simulink model "OPLOOP"  (Simulink 3.00)
settings: Solver=ode45  StartTime=0.0  StopTime=400.0  RelTol=1e-3
libraries: simulink3 x2

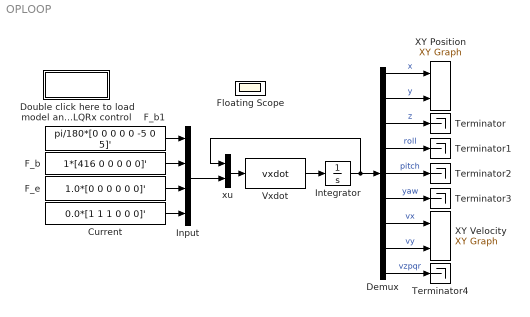
== system OPLOOP ==
  Current : Constant  Value=0.0*[1 1 1 0 0 0]'
  Demux : Demux  Outputs=[1 1 1 1 1 1 1 1 4]
  "Double click here to load model and  LQRx control " : Subsystem
      settings: OpenFcn=shark;global veh;[v1,veh,v3]=vehicle;
      mask Display: disp('Load Data')
  F_b : Constant  Value=1*[416 0 0 0 0 0]'
  F_b1 : Constant  Value=pi/180*[0 0 0 0 0 -5 0 5]'
  F_e : Constant  Value=1.0*[0 0 0 0 0 0]'
  Floating Scope : Scope
      settings: Floating=on  TimeRange=auto  YMin=-1  YMax=1  SaveToWorkspace=off  SaveName=ScopeData  LimitMaxRows=off
  Input : Mux  Inputs=[8 6 6 6]
  Integrator : Integrator  ExternalReset=none  InitialConditionSource=internal  InitialCondition=0  LimitOutput=off  UpperSaturationLimit=inf  LowerSaturationLimit=-inf  ShowSaturationPort=off  ShowStatePort=off  AbsoluteTolerance=auto
  Terminator{,1..4} (5 alike) : Terminator
  Vxdot : MATLABFcn  MATLABFcn=vxdot  OutputWidth=12  OutputSignalType=real
  XY Position : simulink3/Sinks/XY Graph  xmin=0  xmax=16  ymin=-8  ymax=8  st=-1
  XY Velocity : simulink3/Sinks/XY Graph  xmin=-2  xmax=2  ymin=0  ymax=2  st=-1
  xu : Mux  Inputs=[12 26]
  wires:
  Current/1 -> Input/4
  F_b/1 -> Input/2
  F_e/1 -> Input/3
  F_b1/1 -> Input/1
  Input/1 -> xu/2
  xu/1 -> Vxdot/1
  Integrator/1 -> Demux/1, xu/1
  Vxdot/1 -> Integrator/1
  Demux/1 -> XY Position/1  "x"
  Demux/2 -> XY Position/2  "y"
  Demux/4 -> Terminator1/1  "roll"
  Demux/5 -> Terminator2/1  "pitch"
  Demux/6 -> Terminator3/1  "yaw"
  Demux/3 -> Terminator/1  "z"
  Demux/9 -> Terminator4/1  "vzpqr"
  Demux/7 -> XY Velocity/1  "vx"
  Demux/8 -> XY Velocity/2  "vy"

== system OPLOOP/Double click here to load model and  LQRx control  ==
